simulink model "ESP_Model"  (R2018b)
settings: Solver=VariableStepAuto  StartTime=0.0  StopTime=30.0  RelTol=1e-3
settings Model: Creator=patta  LastModifiedBy=patta

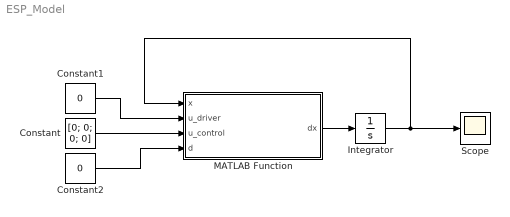
== system ESP_Model ==
  Constant : Constant  Value=[0; 0; 0; 0]
  Constant1 : Constant  Value=0
  Constant2 : Constant  Value=0
  Integrator : Integrator  InitialCondition=[0; 5]
  MATLAB Function : MATLAB Function  TreatAsAtomicUnit=on
  Scope : Scope
  wires:
  MATLAB Function/1(dx) -> Integrator/1
  Integrator/1 -> Scope/1, MATLAB Function/1(x)
  Constant/1 -> MATLAB Function/3(u_control)
  Constant1/1 -> MATLAB Function/2(u_driver)
  Constant2/1 -> MATLAB Function/4(d)

== matlab function ESP_Model/MATLAB Function ==
  data: x input; dx output; u_driver input; u_control input; d input
function dx=Plant(x,u_driver,u_control,d)

g = 9.81; % [m/s^2] gravity acceleration
rho = 1.225; % [kg/m^3] air density
S = 2.4; % [m^2] cross surface
Cx0 = -0.3; % [-] drag coefficient
Cyb = -0.3; % [-] drag coefficient
rk = 1; % dry asphalt
m = 1200; % [kg] vehicle mass
rxf = 1.4;
rxr = -1.6;
ryf = 0.90;
rz =  0.70;
CR = -0.05;
Iz = 1200*(rxr^2+ryf^2)^2;

delta = 0*[1 1 0 0]/180*pi; % 3.5 // 10

rx = [rxf rxf rxr rxr];
ry = [ryf -ryf -ryf ryf];
H = [ones(1,4);
    ry;
    -rx];

%% EQUILIBRIUM POINT

%  global v0 FzW

x0 = 0;
y0 = 0;
v0 = 270/3.6; % [m/s] vehicle speed
beta0 = 0;
w0 = 0;
psi0 = 0/180*pi;
theta = 15/180*pi;

pinvH = pinv(H);
FzW = pinvH*(rz/2*rho*S*v0^2*[0; Cyb*sin(beta0); -Cx0*cos(beta0)]+[m*g*cos(theta); -rz*m*v0*w0*cos(beta0); -rz*m*g*sin(theta)-rz*m*v0*w0*sin(beta0)]);

lambda0s = 0.0061;  %found in main
lambda0 = [lambda0s; lambda0s; 0; 0];

Cf = (FzW(1)+FzW(2))*Partial_mu_long(1,0);
Cr = (FzW(3)+FzW(4))*Partial_mu_long(1,0);
A11 = -(Cf+Cr)/(m*v0);
A12 = -v0-(Cf*rxf+Cr*rxr)/(m*v0);
A21 = -(Cf*rxf+Cr*rxr)/(Iz*v0);
A22 = -(Cf*rxf^2+Cr*rxr^2)/(Iz*v0);
A = [A11 A12
    A21 A22];
B1 = Cf*[1/m;
      rxf/Iz];
B1_Ctrl = ryf/Iz*[zeros(1,4);
             (FzW.').*[-Partial_mu_long(1,lambda0s) Partial_mu_long(1,lambda0s) Partial_mu_long(1,0) -Partial_mu_long(1,0)]];
B2eq = [0; 1/Iz];

dx = A*x+B1*u_driver+B1_Ctrl*u_control;

end

%% Mu

function mu = mu_long(i,lambda)

% 1) Dry asphalt
% 2) wet asphalt
% 3) Snow
% 4) Ice
% 5) Dry Cobblestone
% 6) wet cobblestone
theta1 = [1.28 0.86 0.19 0.05 1.37 0.4];
theta2 = [23.99 33.82 94.13 306.39 6.46 33.71];
theta3 = [0.52 0.35 0.05 0 0.67 0.12];

mu = sign(lambda).*theta1(i).*(1-exp(-abs(lambda)*theta2(i)))-theta3(i)*lambda;

end

%%Partial derivative of mu

function mu = Partial_mu_long(i,lambda)

% 1) Dry asphalt
% 2) wet asphalt
% 3) Snow
% 4) Ice
% 5) Dry Cobblestone
% 6) wet cobblestone
theta1 = [1.28 0.86 0.19 0.05 1.37 0.4];
theta2 = [23.99 33.82 94.13 306.39 6.46 33.71];
theta3 = [0.52 0.35 0.05 0 0.67 0.12];

mu = theta1(i).*theta2(i).*exp(-abs(lambda).*theta2(i))-theta3(i);

end
